simulink model "PathFollower"  (R2019a)
settings: Solver=ode4  StartTime=0.0  StopTime=100  FixedStep=P.Ts  RelTol=1e-3
values from neighbouring files (symbols this model uses):
  desiredPath = [path.flag; path.Va_d; path.r; path.q; path.c; path.rho;     path.lambda]    [main_path_follower.m]
undefined symbols (not defined in the file or in its folder): autopilot, forces_moments, P, path_follower, true_states
libraries: simulink x3
settings Model: Creator=simao  LastModifiedBy=Hugo Pereira

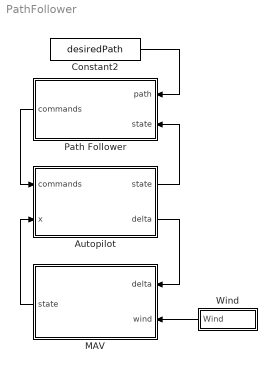
== system PathFollower ==
  Autopilot : Subsystem
      mask Display: image(imread('../autopilot/simulink_imgs/kestrel.jpg'));
  Constant2 : Constant  Value=desiredPath
  MAV : Subsystem
      mask Display: image(imread('../autopilot/simulink_imgs/batcam.png'));
  Path Follower : Subsystem
      mask Display: image(imread('pathFollower_simulink_imgs/pathFollower_mask.png'));
  Wind : Subsystem
  wires:
  Constant2/1 -> Path Follower/1(path)
  Wind/1(Wind) -> MAV/2(wind)
  Autopilot/2(delta) -> MAV/1(delta)
  Autopilot/1(state) -> Path Follower/2(state)
  Path Follower/1(commands) -> Autopilot/1(commands)
  MAV/1(state) -> Autopilot/2(x)

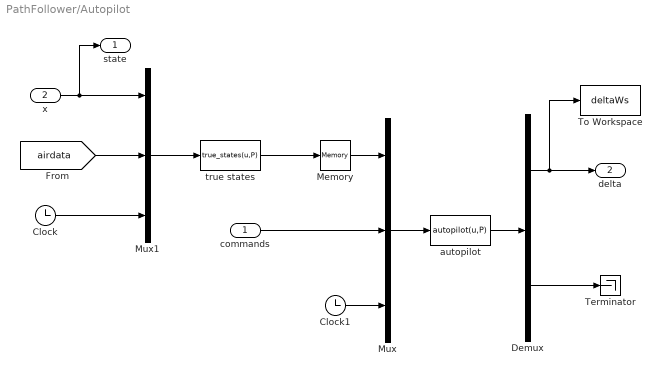
== system PathFollower/Autopilot ==
  commands : Inport
  x : Inport  Port=2
  Clock : Clock
  Clock1 : Clock
  Demux : Demux  Outputs=[4;2]
  Memory : Memory
  Mux : Mux  Inputs=3
  Mux1 : Mux  Inputs=3
  Terminator : Terminator
  To Workspace : ToWorkspace  VariableName=deltaWs  SampleTime=-1
  autopilot : MATLABFcn  MATLABFcn=autopilot(u,P)  OutputDimensions=4+2  SampleTime=P.Ts
  true states : MATLABFcn  MATLABFcn=true_states(u,P)  OutputDimensions=19  SampleTime=P.Ts
  state : Outport
  delta : Outport  Port=2
  wires:
  Mux/1 -> autopilot/1
  Clock/1 -> Mux1/3
  autopilot/1 -> Demux/1
  Demux/1 -> To Workspace/1, delta/1
  Demux/2 -> Terminator/1
  commands/1 -> Mux/2
  Mux1/1 -> true states/1
  x/1 -> state/1, Mux1/1
  true states/1 -> Memory/1
  [airdata] -> Mux1/2
  Memory/1 -> Mux/1
  Clock1/1 -> Mux/3

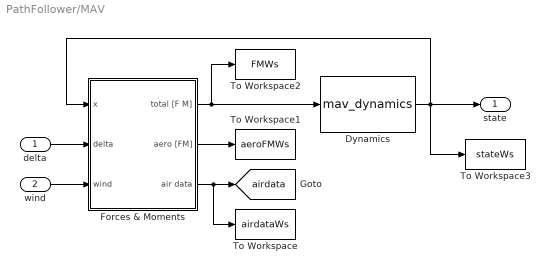
== system PathFollower/MAV ==
  delta : Inport
  wind : Inport  Port=2
  Dynamics : S-Function  FunctionName=mav_dynamics  Parameters=P  SFunctionDeploymentMode=off  EnableBusSupport=off
  Forces & Moments : Subsystem
  To Workspace : ToWorkspace  VariableName=airdataWs  SampleTime=-1
  To Workspace1 : ToWorkspace  VariableName=aeroFMWs  SampleTime=-1
  To Workspace2 : ToWorkspace  VariableName=FMWs  SampleTime=-1
  To Workspace3 : ToWorkspace  VariableName=stateWs  SampleTime=-1
  state : Outport
  tag scope: airdata=global
  wires:
  Dynamics/1 -> To Workspace3/1, state/1, Forces & Moments/1(x)
  Forces & Moments/1(total [F M]) -> To Workspace2/1, Dynamics/1
  Forces & Moments/3(air data) -> [airdata], To Workspace/1
  delta/1 -> Forces & Moments/2(delta)
  wind/1 -> Forces & Moments/3(wind)
  Forces & Moments/2(aero [FM]) -> To Workspace1/1

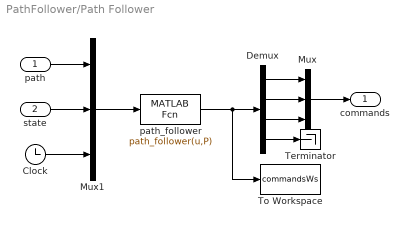
== system PathFollower/Path Follower ==
  path : Inport
  state : Inport  Port=2
  Clock : Clock
  Demux : Demux
  Mux : Mux  Inputs=3
  Mux1 : Mux  Inputs=3
  Terminator : Terminator
  To Workspace : ToWorkspace  VariableName=commandsWs  SampleTime=-1
  path_follower : MATLABFcn  MATLABFcn=path_follower(u,P)  OutputDimensions=4  SampleTime=5*P.Ts
  commands : Outport
  wires:
  Demux/1 -> Mux/1
  Demux/2 -> Mux/2
  Demux/3 -> Mux/3
  Demux/4 -> Terminator/1
  Mux/1 -> commands/1
  state/1 -> Mux1/2
  Mux1/1 -> path_follower/1
  path/1 -> Mux1/1
  Clock/1 -> Mux1/3
  path_follower/1 -> To Workspace/1, Demux/1

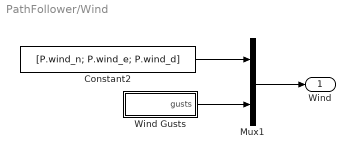
== system PathFollower/Wind ==
  Constant2 : Constant  Value=[P.wind_n; P.wind_e; P.wind_d]
  Mux1 : Mux  Inputs=2
  Wind Gusts : Subsystem
  Wind : Outport
  wires:
  Constant2/1 -> Mux1/1
  Mux1/1 -> Wind/1
  Wind Gusts/1(gusts) -> Mux1/2

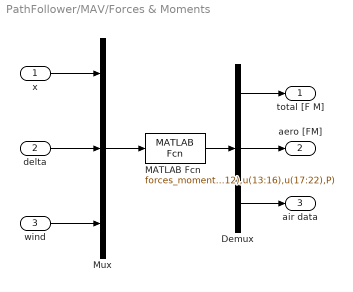
== system PathFollower/MAV/Forces & Moments ==
  x : Inport
  delta : Inport  Port=2
  wind : Inport  Port=3
  Demux : Demux  Outputs=[6;6;7]
  MATLAB Fcn : MATLABFcn  MATLABFcn=forces_moments(u(1:12),u(13:16),u(17:22),P)  OutputDimensions=19
  Mux : Mux  Inputs=3
  total [F M] : Outport
  aero [FM] : Outport  Port=2
  air data : Outport  Port=3
  wires:
  Mux/1 -> MATLAB Fcn/1
  Demux/1 -> total [F M]/1
  MATLAB Fcn/1 -> Demux/1
  wind/1 -> Mux/3
  delta/1 -> Mux/2
  x/1 -> Mux/1
  Demux/3 -> air data/1
  Demux/2 -> aero [FM]/1

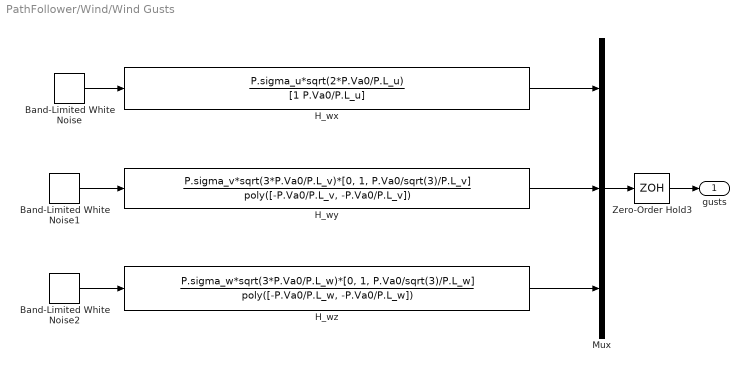
== system PathFollower/Wind/Wind Gusts ==
  Band-Limited White Noise : simulink/Sources/Band-Limited White Noise  Cov=[1]  Ts=P.Ts  seed=[23341]
  Band-Limited White Noise1 : simulink/Sources/Band-Limited White Noise  Cov=[1]  Ts=P.Ts  seed=[23341]
  Band-Limited White Noise2 : simulink/Sources/Band-Limited White Noise  Cov=[1]  Ts=P.Ts  seed=[23341]
  H_wx : TransferFcn  Numerator=P.sigma_u*sqrt(2*P.Va0/P.L_u)  Denominator=[1 P.Va0/P.L_u]
  H_wy : TransferFcn  Numerator=P.sigma_v*sqrt(3*P.Va0/P.L_v)*[0, 1, P.Va0/sqrt(3)/P.L_v]  Denominator=poly([-P.Va0/P.L_v, -P.Va0/P.L_v])
  H_wz : TransferFcn  Numerator=P.sigma_w*sqrt(3*P.Va0/P.L_w)*[0, 1, P.Va0/sqrt(3)/P.L_w]  Denominator=poly([-P.Va0/P.L_w, -P.Va0/P.L_w])
  Mux : Mux  Inputs=3
  Zero-Order Hold3 : ZeroOrderHold  SampleTime=P.Ts
  gusts : Outport
  wires:
  H_wx/1 -> Mux/1
  Band-Limited White Noise/1 -> H_wx/1
  H_wy/1 -> Mux/2
  Band-Limited White Noise1/1 -> H_wy/1
  H_wz/1 -> Mux/3
  Band-Limited White Noise2/1 -> H_wz/1
  Mux/1 -> Zero-Order Hold3/1
  Zero-Order Hold3/1 -> gusts/1
